simulink model "Kalman_Modular_Simple"  (R2019b)
settings: Solver=VariableStepAuto  StartTime=0.0  StopTime=phase_ns_model.sim_dur  FixedStep=model.Ts  RelTol=1e-6
undefined symbols (not defined in the file or in its folder): phase_ns_model
libraries: dspsrcs4 x4
settings Model: Creator=isidoraradenkovic  LastModifiedBy=isidoraradenkovic

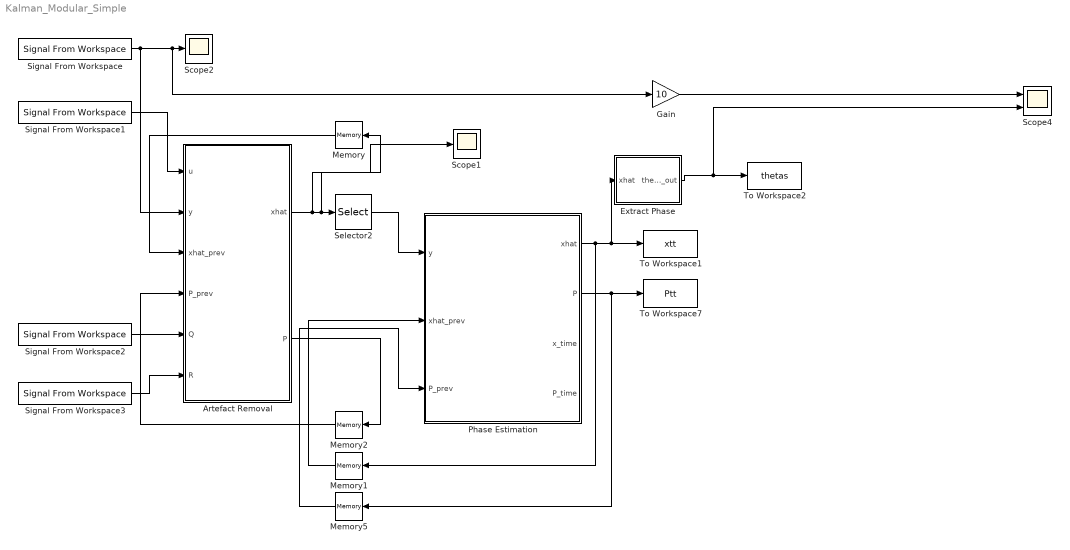
== system Kalman_Modular_Simple ==
  Artefact Removal : MATLAB Function  TreatAsAtomicUnit=on
  Extract Phase : MATLAB Function  TreatAsAtomicUnit=on
  Gain : Gain  Gain=10
  Memory : Memory  InitialCondition=[0; 0]  InheritSampleTime=on
  Memory1 : Memory  InitialCondition=[0; 0]  InheritSampleTime=on
  Memory2 : Memory  InitialCondition=[0 0; 0 0]  InheritSampleTime=on
  Memory5 : Memory  InitialCondition=[0 0; 0 0]  InheritSampleTime=on
  Phase Estimation : MATLAB Function  TreatAsAtomicUnit=on
  Scope1 : Scope
  Scope2 : Scope
  Scope4 : Scope  NumInputPorts=2
  Selector2 : Selector  InputPortWidth=2  IndexOptions=Index vector (dialog)  Indices=[1]  OutputSizes=1
  Signal From Workspace : dspsrcs4/Signal From Workspace  X=input_data  Ts=phase_ns_model.Ts  nsamps=1  OutputAfterFinalValue=Cyclic repetition  ignoreOrWarnInputAndFrameLengths=off  OutputFrames=off
  Signal From Workspace1 : dspsrcs4/Signal From Workspace  X=tms_pulses  Ts=phase_ns_model.Ts  nsamps=1  OutputAfterFinalValue=Cyclic repetition  ignoreOrWarnInputAndFrameLengths=off  OutputFrames=off
  Signal From Workspace2 : dspsrcs4/Signal From Workspace  X=phase_ns_model.Q1  Ts=phase_ns_model.Ts/2  nsamps=2  OutputAfterFinalValue=Cyclic repetition  ignoreOrWarnInputAndFrameLengths=off  OutputFrames=off
  Signal From Workspace3 : dspsrcs4/Signal From Workspace  X=phase_double_model.R  Ts=phase_ns_model.Ts  nsamps=1  OutputAfterFinalValue=Cyclic repetition  ignoreOrWarnInputAndFrameLengths=off  OutputFrames=off
  To Workspace1 : ToWorkspace  VariableName=xtt  SampleTime=-1
      settings: Save2DSignal=2-D array (concatenate along first dimension)
  To Workspace2 : ToWorkspace  VariableName=thetas  SampleTime=-1
      settings: Save2DSignal=2-D array (concatenate along first dimension)
  To Workspace7 : ToWorkspace  VariableName=Ptt  SampleTime=-1
      settings: Save2DSignal=2-D array (concatenate along first dimension)
  wires:
  Signal From Workspace1/1 -> Artefact Removal/1(u)
  Signal From Workspace/1 -> Artefact Removal/2(y), Gain/1, Scope2/1
  Phase Estimation/2(P) -> To Workspace7/1, Memory5/1
  Artefact Removal/1(xhat) -> Memory/1, Scope1/1, Selector2/1
  Extract Phase/1(thetas_out) -> Scope4/2, To Workspace2/1
  Memory2/1 -> Artefact Removal/4(P_prev)
  Memory1/1 -> Phase Estimation/2(xhat_prev)
  Memory5/1 -> Phase Estimation/3(P_prev)
  Memory/1 -> Artefact Removal/3(xhat_prev)
  Phase Estimation/1(xhat) -> Extract Phase/1(xhat), To Workspace1/1, Memory1/1
  Artefact Removal/2(P) -> Memory2/1
  Signal From Workspace2/1 -> Artefact Removal/5(Q)
  Selector2/1 -> Phase Estimation/1(y)
  Signal From Workspace3/1 -> Artefact Removal/6(R)
  Gain/1 -> Scope4/1

== matlab function Kalman_Modular_Simple/Phase Estimation ==
  data: xhat output; y input; xhat_prev input; P_prev input; P output; x_time output; P_time output; phase_ns_model parameter
function [xhat, P, x_time, P_time] = phase_kalman(y, xhat_prev, P_prev, phase_ns_model)
x_time = phase_ns_model.A*xhat_prev;
P_time = phase_ns_model.A*P_prev*phase_ns_model.A'+ phase_ns_model.Q2;

K = P_time*(phase_ns_model.C')*pinv(phase_ns_model.C*P_time*phase_ns_model.C' + phase_ns_model.R2);
epsilon = y - phase_ns_model.C*x_time;

xhat = x_time + K*epsilon;
P = P_time - K*phase_ns_model.C*P_time;
end

== matlab function Kalman_Modular_Simple/Extract Phase ==
  settings: sampleTime=combined_model.Ts
  data: xhat input; thetas_out output; phase_ns_model parameter
function thetas_out  = extract_phase(xhat, phase_ns_model)

thetas_out = mod(atan2(xhat(2), xhat(1)) - pi/2 - 2*pi*phase_ns_model.Ts*phase_ns_model.f, 2*pi)-pi;
%thetas_out = atan2(xhat(2), xhat(1));

== matlab function Kalman_Modular_Simple/Artefact Removal ==
  data: u input; xhat output; y input; xhat_prev input; P_prev input; Q input; R input; P output; phase_double_model parameter
function [xhat, P] = artefact_kalman(u, y, xhat_prev, P_prev, Q, R, phase_double_model)
x_time = phase_double_model.A*xhat_prev + phase_double_model.B*u;
P_time = phase_double_model.A*P_prev*phase_double_model.A'+ Q;

K = P_time*(phase_double_model.C')*pinv(phase_double_model.C*P_time*phase_double_model.C' + R);
epsilon = y - phase_double_model.C*x_time;

xhat = x_time + K*epsilon;
P = P_time - K*phase_double_model.C*P_time;
